simulink model "watchIF"  (Simulink 8.2)
settings: Solver=ode45  StartTime=0.0  StopTime=Inf  RelTol=1e-3
libraries: simulink x5
settings Model: Creator=Marco  LastModifiedBy=Marco

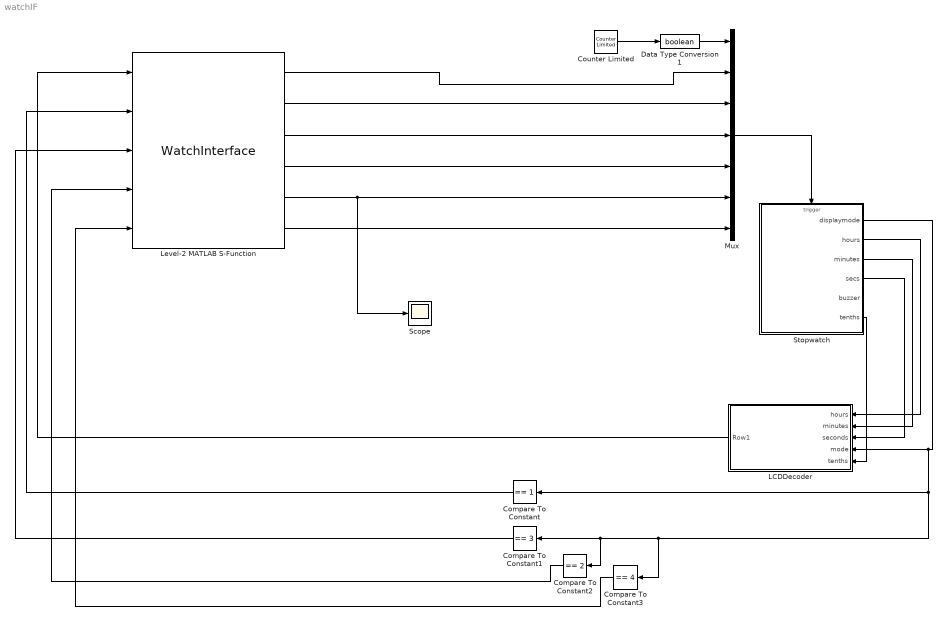
== system watchIF ==
  Compare To Constant : simulink/Logic and Bit Operations/Compare To Constant  relop===  const=1  OutDataTypeStr=boolean
  Compare To Constant1 : simulink/Logic and Bit Operations/Compare To Constant  relop===  const=3  OutDataTypeStr=boolean
  Compare To Constant2 : simulink/Logic and Bit Operations/Compare To Constant  relop===  const=2  OutDataTypeStr=boolean
  Compare To Constant3 : simulink/Logic and Bit Operations/Compare To Constant  relop===  const=4  OutDataTypeStr=boolean
  Counter Limited : simulink/Sources/Counter Limited  uplimit=1  tsamp=0.1
  Data Type Conversion1 : DataTypeConversion  OutDataTypeStr=boolean
  LCDDecoder : Subsystem
  Level-2 MATLAB S-Function : M-S-Function  FunctionName=WatchInterface
  Mux : Mux  Inputs=7
  Scope : Scope
  Stopwatch : Stateflow chart  TreatAsAtomicUnit=on
  wires:
  Mux/1 -> Stopwatch/Trigger
  Stopwatch/2(hours) -> LCDDecoder/1(hours)
  Stopwatch/3(minutes) -> LCDDecoder/2(minutes)
  Stopwatch/4(secs) -> LCDDecoder/3(seconds)
  Stopwatch/1(displaymode) -> Compare To Constant3/1, Compare To Constant2/1, Compare To Constant1/1, Compare To Constant/1, LCDDecoder/4(mode)
  Data Type Conversion1/1 -> Mux/1
  Stopwatch/6(tenths) -> LCDDecoder/5(tenths)
  Counter Limited/1 -> Data Type Conversion1/1
  LCDDecoder/1(Row1) -> Level-2 MATLAB S-Function/1
  Compare To Constant/1 -> Level-2 MATLAB S-Function/2
  Compare To Constant1/1 -> Level-2 MATLAB S-Function/3
  Level-2 MATLAB S-Function/1 -> Mux/2
  Level-2 MATLAB S-Function/2 -> Mux/3
  Level-2 MATLAB S-Function/3 -> Mux/4
  Level-2 MATLAB S-Function/4 -> Mux/5
  Level-2 MATLAB S-Function/5 -> Scope/1, Mux/6
  Level-2 MATLAB S-Function/6 -> Mux/7
  Compare To Constant2/1 -> Level-2 MATLAB S-Function/4
  Compare To Constant3/1 -> Level-2 MATLAB S-Function/5

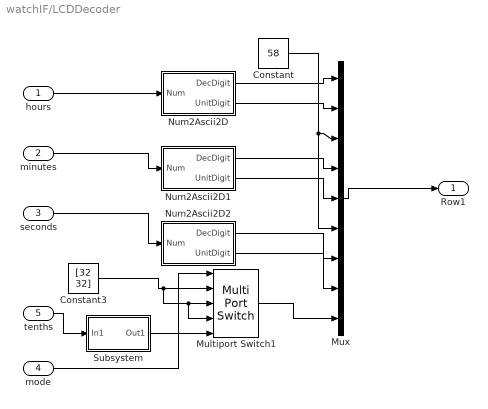
== system watchIF/LCDDecoder ==
  hours : Inport
  minutes : Inport  Port=2
  seconds : Inport  Port=3
  mode : Inport  Port=4
  tenths : Inport  Port=5
  Constant : Constant  Value=58  OutDataTypeStr=uint8
  Constant3 : Constant  Value=[32 32]  OutDataTypeStr=uint8
  Multiport Switch1 : MultiPortSwitch  Inputs=4  DiagnosticForDefault=None
  Mux : Mux  Inputs=9
  Num2Ascii2D : Subsystem
  Num2Ascii2D1 : Subsystem
  Num2Ascii2D2 : Subsystem
  Subsystem : Subsystem
  Row1 : Outport
  wires:
  hours/1 -> Num2Ascii2D/1(Num)
  minutes/1 -> Num2Ascii2D1/1(Num)
  seconds/1 -> Num2Ascii2D2/1(Num)
  Mux/1 -> Row1/1
  Constant/1 -> Mux/3, Mux/6
  Num2Ascii2D/1(DecDigit) -> Mux/1
  Num2Ascii2D/2(UnitDigit) -> Mux/2
  Num2Ascii2D1/1(DecDigit) -> Mux/4
  Num2Ascii2D1/2(UnitDigit) -> Mux/5
  Num2Ascii2D2/1(DecDigit) -> Mux/7
  Num2Ascii2D2/2(UnitDigit) -> Mux/8
  mode/1 -> Multiport Switch1/1
  Multiport Switch1/1 -> Mux/9
  Subsystem/1(Out1) -> Multiport Switch1/5
  tenths/1 -> Subsystem/1(In1)
  Constant3/1 -> Multiport Switch1/2, Multiport Switch1/3, Multiport Switch1/4

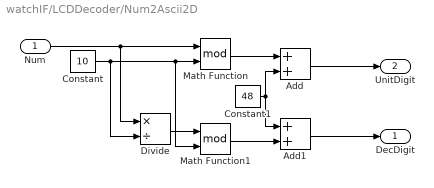
== system watchIF/LCDDecoder/Num2Ascii2D ==
  Num : Inport
  Add : Sum
  Add1 : Sum
  Constant : Constant  Value=10  OutDataTypeStr=uint8
  Constant1 : Constant  Value=48  OutDataTypeStr=uint8
  Divide : Product  Inputs=*/  OutDataTypeStr=uint8
  Math Function : Math  Operator=mod  SaturateOnIntegerOverflow=on
  Math Function1 : Math  Operator=mod  SaturateOnIntegerOverflow=on
  DecDigit : Outport
  UnitDigit : Outport  Port=2
  wires:
  Num/1 -> Math Function/1, Divide/1
  Constant/1 -> Divide/2, Math Function/2, Math Function1/2
  Divide/1 -> Math Function1/1
  Math Function/1 -> Add/1
  Add/1 -> UnitDigit/1
  Add1/1 -> DecDigit/1
  Math Function1/1 -> Add1/2
  Constant1/1 -> Add/2, Add1/1

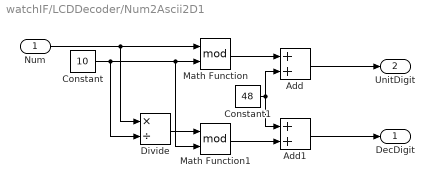
== system watchIF/LCDDecoder/Num2Ascii2D1 ==
  Num : Inport
  Add : Sum
  Add1 : Sum
  Constant : Constant  Value=10  OutDataTypeStr=uint8
  Constant1 : Constant  Value=48  OutDataTypeStr=uint8
  Divide : Product  Inputs=*/  OutDataTypeStr=uint8
  Math Function : Math  Operator=mod  SaturateOnIntegerOverflow=on
  Math Function1 : Math  Operator=mod  SaturateOnIntegerOverflow=on
  DecDigit : Outport
  UnitDigit : Outport  Port=2
  wires:
  Num/1 -> Math Function/1, Divide/1
  Constant/1 -> Divide/2, Math Function/2, Math Function1/2
  Divide/1 -> Math Function1/1
  Math Function/1 -> Add/1
  Add/1 -> UnitDigit/1
  Add1/1 -> DecDigit/1
  Math Function1/1 -> Add1/2
  Constant1/1 -> Add/2, Add1/1

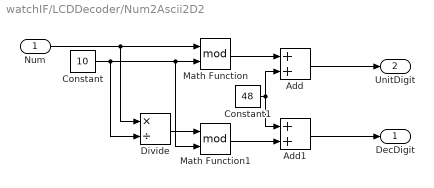
== system watchIF/LCDDecoder/Num2Ascii2D2 ==
  Num : Inport
  Add : Sum
  Add1 : Sum
  Constant : Constant  Value=10  OutDataTypeStr=uint8
  Constant1 : Constant  Value=48  OutDataTypeStr=uint8
  Divide : Product  Inputs=*/  OutDataTypeStr=uint8
  Math Function : Math  Operator=mod  SaturateOnIntegerOverflow=on
  Math Function1 : Math  Operator=mod  SaturateOnIntegerOverflow=on
  DecDigit : Outport
  UnitDigit : Outport  Port=2
  wires:
  Num/1 -> Math Function/1, Divide/1
  Constant/1 -> Divide/2, Math Function/2, Math Function1/2
  Divide/1 -> Math Function1/1
  Math Function/1 -> Add/1
  Add/1 -> UnitDigit/1
  Add1/1 -> DecDigit/1
  Math Function1/1 -> Add1/2
  Constant1/1 -> Add/2, Add1/1

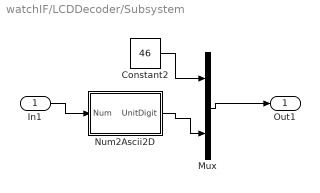
== system watchIF/LCDDecoder/Subsystem ==
  In1 : Inport
  Constant2 : Constant  Value=46  OutDataTypeStr=uint8
  Mux : Mux  Inputs=2
  Num2Ascii2D : Subsystem
  Out1 : Outport
  wires:
  Constant2/1 -> Mux/1
  Num2Ascii2D/1(UnitDigit) -> Mux/2
  In1/1 -> Num2Ascii2D/1(Num)
  Mux/1 -> Out1/1

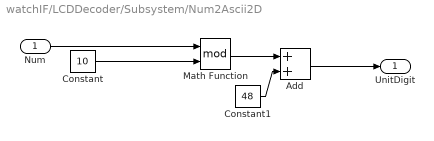
== system watchIF/LCDDecoder/Subsystem/Num2Ascii2D ==
  Num : Inport
  Add : Sum
  Constant : Constant  Value=10  OutDataTypeStr=uint8
  Constant1 : Constant  Value=48  OutDataTypeStr=uint8
  Math Function : Math  Operator=mod  SaturateOnIntegerOverflow=on
  UnitDigit : Outport
  wires:
  Num/1 -> Math Function/1
  Constant/1 -> Math Function/2
  Math Function/1 -> Add/1
  Add/1 -> UnitDigit/1
  Constant1/1 -> Add/2

== stateflow chart Stopwatch ==
  state control [parallel]
    settings: executionOrder=2
    state stopwatch
      en:displaymode=4
      state stop
      (default) -> stop
    state timeset
      en:displaymode=3
      state sethours
        en:hours=Thours
      (default) -> control.timeset.sethours : /hours=Thours;minutes=Tminutes;secs=0
      control.timeset.sethours -> control.timeset.sethours [order 2] : buttonP/Thours=(Thours+1)%%24
      control.timeset.sethours -> control.timeset.sethours [order 1] : buttonM[Thours==0]/Thours=23
      control.timeset.sethours -> control.timeset.sethours [order 3] : buttonM/Thours=Thours-1
    state time
      en:displaymode=1
      control.time -> control.time [order 1] : tens/hours=Thours;minutes=Tminutes;secs=Tseconds
    state alarmset
      en: displaymode=2
      state sethours
        en:hours=Ahours
      (default) -> control.alarmset.sethours : /hours=Ahours;minutes=Aminutes;secs=0
      control.alarmset.sethours -> control.alarmset.sethours [order 2] : buttonP/Ahours=(Ahours+1)%%24
      control.alarmset.sethours -> control.alarmset.sethours [order 3] : buttonM/Ahours=Ahours-1
      control.alarmset.sethours -> control.alarmset.sethours [order 1] : buttonM[Ahours==0]/Ahours=23
    control -> control.time : timemode
    (default) -> control.time : /Ahours=0; Aminutes=0;
    control.time -> alarmset [order 1] : alarmsetmode
    stopwatch -> alarmset [order 1] : alarmsetmode
    alarmset -> stopwatch [order 2] : swatchsetmode
    alarmset -> timeset [order 1] : timesetmode/timeseton
    timeset -> alarmset [order 2] : alarmsetmode
    control.time -> stopwatch [order 2] : swatchsetmode
    control.time -> timeset [order 3] : timesetmode
    timeset -> stopwatch [order 1] : swatchsetmode
    stopwatch -> timeset [order 2] : timesetmode
  state buzzer [parallel]
    settings: executionOrder=3
    state off
      en:buzzer=0
    (default) -> off
  state time [parallel]
    settings: executionOrder=1
    state ticking
    state setup
    (default) -> ticking : /Thours=0; Tminutes=0; Tseconds=0; Ttens=0
    ticking -> (junction 38) [order 2] : tens{Ttens=(Ttens+1)%%10}
    (junction 38) -> (junction 39) : [Ttens==0]{Tseconds=(Tseconds+1)%%60}
    (junction 40) -> ticking : [Tminutes==0]/Thours=(Thours+1)%%24
    setup -> ticking : timeseton
    ticking -> setup [order 1] : timeseton
    (junction 39) -> (junction 40) : [Tseconds==0]/Tminutes=(Tminutes+1)%%60
  data: displaymode output uint8; Thours local uint8; Tminutes local uint8; Tseconds local uint8; Ahours local uint8; Aminutes local uint8; hours output uint8; minutes output uint8; secs output uint8; buzzer output boolean; Chours local uint8; Cminutes local uint8; Cseconds local uint8; tenths output uint8; Ttens local uint8
  events: tens input EITHER_EDGE_EVENT; timemode input RISING_EDGE_EVENT; timesetmode input RISING_EDGE_EVENT; alarmsetmode input RISING_EDGE_EVENT; swatchsetmode input RISING_EDGE_EVENT; buttonP input RISING_EDGE_EVENT; timeseton local EITHER_EDGE_EVENT; buttonM input RISING_EDGE_EVENT
